simulink model "Accelrator"  (R2023a)
settings: Solver=VariableStepAuto  StartTime=0.0  StopTime=10.0  RelTol=1e-3
settings Model: Creator=Egypt_Laptop  LastModifiedBy=Egypt_Laptop

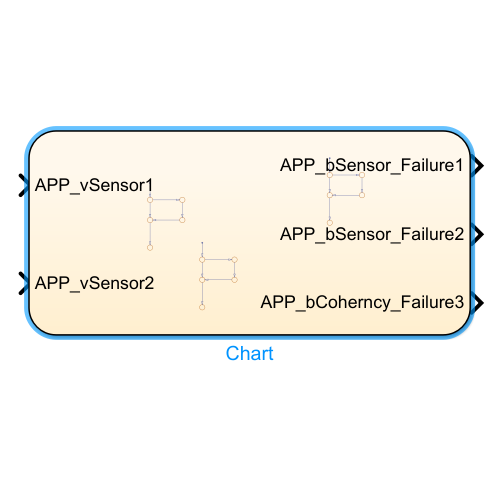
[thumbnail: Simulink's stored preview of the top-level diagram]
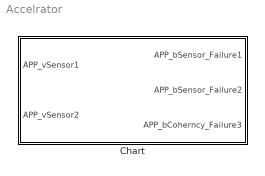
== system Accelrator ==
  Chart : Stateflow chart  TreatAsAtomicUnit=on

== stateflow chart Accelrator/Chart ==
  (default) -> (junction 12) : /* Sensor1 */
  (junction 12) -> (junction 13) [order 1] : [APP_vSensor1>4.5 || APP_vSensor1 <0.5]
  (junction 12) -> (junction 14) [order 2] : {APP_bSensor_Failure1 = 0;}
  (junction 13) -> (junction 15) : {APP_bSensor_Failure1 = 1;}
  (junction 15) -> (junction 14)
  (junction 14) -> (junction 70)
  (junction 70) -> (junction 72) [order 1] : [APP_vSensor2>4.5 || APP_vSensor2 <0.5]
  (junction 70) -> (junction 71) [order 2] : {APP_bSensor_Failure2 = 0;}
  (junction 72) -> (junction 73) : {APP_bSensor_Failure2 = 1;}
  (junction 73) -> (junction 71)
  (junction 71) -> (junction 51)
  (junction 51) -> (junction 43) [order 1] : [(APP_vSensor1 + APP_vSensor2) != 5]
  (junction 51) -> (junction 52) [order 2] : {APP_bCoherncy_Failure3 = 0;}
  (junction 43) -> (junction 47) : {APP_bCoherncy_Failure3 = 1;}
  (junction 47) -> (junction 52)
  (junction 52) -> (junction 45)
  data: APP_vSensor1 input double; APP_vSensor2 input double; APP_bSensor_Failure1 output double; APP_bSensor_Failure2 output double; APP_bCoherncy_Failure3 output double
